simulink model "Simulink_carrillo"  (R2024a)
settings: Solver=VariableStepAuto  StartTime=0.0  StopTime=5  RelTol=1e-3
values from neighbouring files (symbols this model uses):
  b1 = 1000    [Datos_Simu.m]    (also in Ec2.m)
  k1 = 16182    [Datos_Simu.m]    (also in Ec2.m)
  k2 = 19000    [Datos_Simu.m]    (also in Ec2.m)
  m1 = 290    [Datos_Simu.m]    (also in Ec2.m)
  m2 = 59    [Datos_Simu.m]    (also in Ec2.m)
settings Model: Creator=Braulio Ramíreza  LastModifiedBy=Braulio Ramíreza

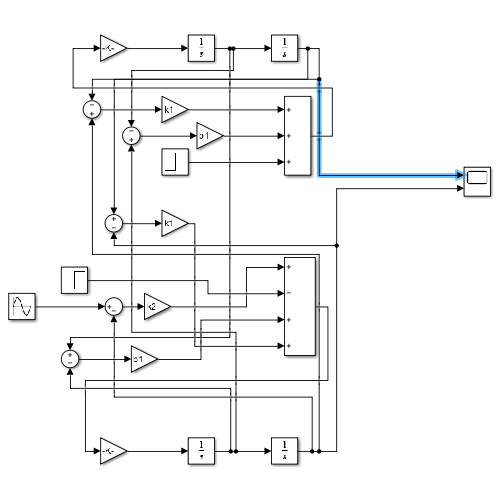
[thumbnail: Simulink's stored preview of the top-level diagram]
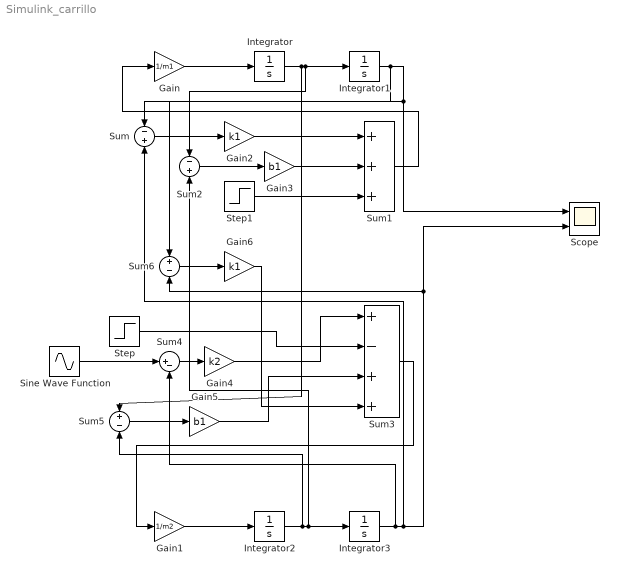
== system Simulink_carrillo ==
  Gain : Gain  Gain=1/m1
  Gain1 : Gain  Gain=1/m2
  Gain2 : Gain  Gain=k1
  Gain3 : Gain  Gain=b1
  Gain4 : Gain  Gain=k2
  Gain5 : Gain  Gain=b1
  Gain6 : Gain  Gain=k1
  Integrator{,1..3} (4 alike) : Integrator
  Scope : Scope  NumInputPorts=2
  Sine Wave Function : Sin  Amplitude=0.05  Frequency=0.5*pi  SampleTime=0
  Step : Step  Time=0  After=0  SampleTime=0
  Step1 : Step  Time=0  After=0  SampleTime=0
  Sum : Sum  Inputs=-+
  Sum1 : Sum  Inputs=+++
  Sum2 : Sum  Inputs=-+
  Sum3 : Sum  Inputs=+-++
  Sum4 : Sum  Inputs=|+-
  Sum5 : Sum  Inputs=+-
  Sum6 : Sum  Inputs=+-
  wires:
  Integrator/1 -> Integrator1/1, Sum2/1, Sum5/1
  Gain/1 -> Integrator/1
  Gain1/1 -> Integrator2/1
  Integrator2/1 -> Sum5/2, Integrator3/1, Sum2/2
  Integrator1/1 -> Sum6/1, Scope/1, Sum/1
  Integrator3/1 -> Sum4/2, Scope/2, Sum6/2, Sum/2
  Sum/1 -> Gain2/1
  Gain2/1 -> Sum1/1
  Sum2/1 -> Gain3/1
  Gain3/1 -> Sum1/2
  Step1/1 -> Sum1/3
  Sum1/1 -> Gain/1
  Sine Wave Function/1 -> Sum4/1
  Step/1 -> Sum3/2
  Sum4/1 -> Gain4/1
  Gain4/1 -> Sum3/1
  Sum5/1 -> Gain5/1
  Gain5/1 -> Sum3/3
  Sum6/1 -> Gain6/1
  Gain6/1 -> Sum3/4
  Sum3/1 -> Gain1/1
